simulink model "deadReckoning_rover_closedloop_mc40"  (R2023a)
settings: Solver=FixedStepAuto  StartTime=0.0  StopTime=inf  FixedStep=0.01  RelTol=1e-3  EnableMultiTasking=on
PreLoadFcn:
  | robotParameters;
model workspace (MAT data in the model file):
  axleLength = 0.085
  ticksPerRot = 1200
  wheelR = 0.045
undefined symbols (not defined in the file): DiscIntNeverNeededParam
libraries: M5Core_Library x4, simulink x1
settings Model: ExtModeTrigDuration=2  Creator=sseshadr  LastModifiedBy=auw_a
settings SolverCC: AlgebraicLoopSolver=TrustRegion
settings DataIOCC: ReturnWorkspaceOutputs=off
settings OptimizationCC: MaxStackSize=64  EfficientTunableParamExpr=on
settings DebuggingCC: ParameterPrecisionLossMsg=none  ParameterTunabilityLossMsg=error  UnconnectedInputMsg=warning  UnconnectedOutputMsg=warning  UnconnectedLineMsg=warning  ArithmeticOperatorsInVariantConditions=warning
settings HardwareCC: ProdBitPerPointer=32  ProdBitPerSizeT=32  ProdBitPerPtrDiffT=32  ProdLargestAtomicInteger=Long  ProdLargestAtomicFloat=Double  ProdWordSize=32  ProdHWDeviceType=ARM Compatible->ARM Cortex
settings ModelReferenceCC: EnableRefExpFcnMdlSchedulingChecks=on
settings SFSimCC: SimUseLocalCustomCode=off  MATLABDynamicMemAlloc=off  CustomCodeUndefinedFunction=UseInterfaceOnly
settings RTWCC: Description=Embedded Coder  SystemTargetFile=ert.tlc  HardwareBoard=ESP32-WROOM(Arduino Compatible)  TLCOptions="-aInlineSetEventsForThisBaseRateFcn=TLC_FALSE -aSuppressMultiTaskScheduler=TLC_FALSE    -aRateBasedStepFcn=0"  TemplateMakefile=ert_default_tmf  GenerateReport=on  RTWUseLocalCustomCode=off  Toolchain=ESP32  BuildConfiguration=Faster Runs  IncludeHyperlinkInReport=on  GenerateTraceInfo=on  GenerateTraceReport=on  GenerateTraceReportSl=on  GenerateTraceReportSf=on  GenerateTraceReportEml=on  DLArmComputeVersion=19.05
settings CodeAppCC: ForceParamTrailComments=on  IgnoreCustomStorageClasses=off  OperatorAnnotations=on  SimulinkDataObjDesc=on  SFDataObjDesc=on  MATLABFcnDesc=on  InsertBlockDesc=on  StateflowObjectComments=on  MATLABSourceComments=on
settings ERTTargetCC: MultiwordLength=2048  SupportContinuousTime=on  SupportVariableSizeSignals=on  ExtModeTransport=2  ExtModeStaticAlloc=on  ExtModeAutomaticAllocSize=off  ExtModeStaticAllocSize=65536  ExtModeMexFile=ext_xcp  ExtModeIntrfLevel=Level2 - Open

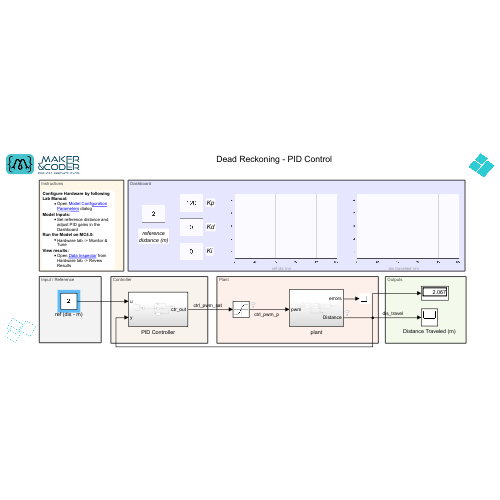
[thumbnail: Simulink's stored preview of the top-level diagram]
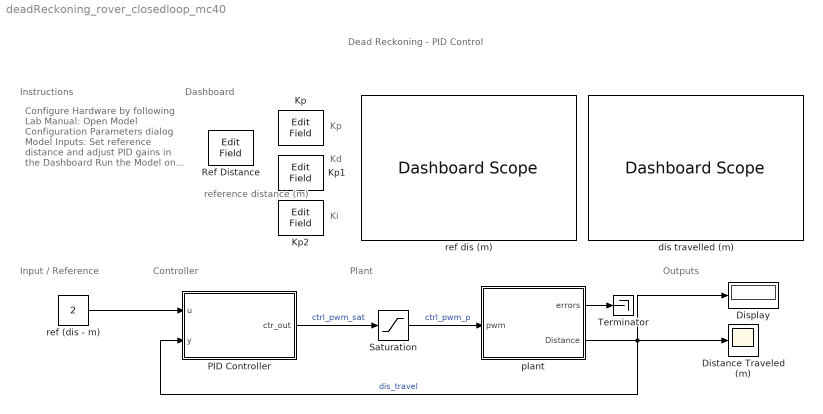
== system deadReckoning_rover_closedloop_mc40 ==
  note: Kp
  note: reference
      | distance (m)
  note: Dashboard
  note: Outputs
  note: Plant
  note: Controller
  note: Input / Reference
  note: Dead Reckoning - PID Control
  note: Kd
  note: Ki
  note: Configure Hardware by following Lab Manual:
      | Open Model Configuration Parameters dialog
      | Model Inputs:
      | Set reference distance and adjust PID gains in the Dashboard
      | Run the Model on MC4.0:
      | Hardware tab -> Monitor & Tune
      | View results:
      | Open Data Inspector from Hardware tab -> Revew Results
  note: Instructions
  Display : Display
  Distance Traveled (m) : Scope
  Kp : EditField  LabelPosition=Hide  ShowInitialText=on  Alignment=Center
  Kp1 : EditField  LabelPosition=Hide  ShowInitialText=on  Alignment=Center
  Kp2 : EditField  LabelPosition=Hide  ShowInitialText=on  Alignment=Center
  PID Controller : Subsystem
  Ref Distance : EditField  LabelPosition=Hide  ShowInitialText=on  Alignment=Center
  Saturation : Saturate  UpperLimit=127  LowerLimit=-127
  Terminator : Terminator
  dis travelled (m) : DashboardScope  Ymin=-5  Ymax=5  UpdateMode=Scroll
  plant : Subsystem
  ref (dis - m) : Constant  Value=2
  ref dis (m) : DashboardScope  Ymin=-5  Ymax=5  UpdateMode=Scroll
  wires:
  Saturation/1 -> plant/1(pwm)  "ctrl_pwm_p"
  plant/2(Distance) -> PID Controller/2(y), Distance Traveled (m)/1, Display/1  "dis_travel"
  ref (dis - m)/1 -> PID Controller/1(u)
  plant/1(errors) -> Terminator/1
  PID Controller/1(ctr_out) -> Saturation/1  "ctrl_pwm_sat"

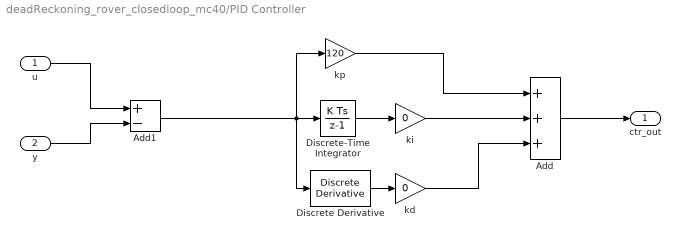
== system deadReckoning_rover_closedloop_mc40/PID Controller ==
  u : Inport
  y : Inport  Port=2
  Add : Sum  Inputs=+++
  Add1 : Sum  Inputs=+-
  Discrete Derivative : simulink/Discrete/Discrete Derivative  gainval=1.0  ICPrevScaledInput=0.0  OutMin=[]  OutMax=[]  OutDataType=fixdt(1, 16)  OutScaling=2^-10  DoSatur=off
  Discrete-Time Integrator : DiscreteIntegrator  SampleTime=-1  ICPrevOutput=DiscIntNeverNeededParam  ICPrevScaledInput=DiscIntNeverNeededParam
  kd : Gain  Gain=0
  ki : Gain  Gain=0
  kp : Gain  Gain=120
  ctr_out : Outport
  wires:
  kp/1 -> Add/1
  kd/1 -> Add/3
  Discrete-Time Integrator/1 -> ki/1
  Add1/1 -> Discrete Derivative/1, Discrete-Time Integrator/1, kp/1
  Discrete Derivative/1 -> kd/1
  ki/1 -> Add/2
  Add/1 -> ctr_out/1
  u/1 -> Add1/1
  y/1 -> Add1/2

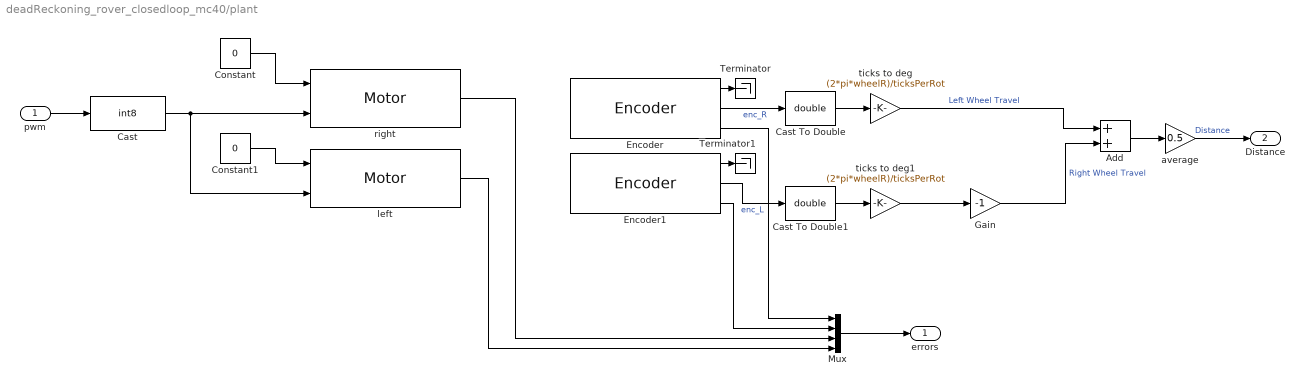
== system deadReckoning_rover_closedloop_mc40/plant ==
  pwm : Inport
  Add : Sum
  Cast : DataTypeConversion  OutDataTypeStr=int8  SaturateOnIntegerOverflow=off  RndMeth=Floor
  Cast To Double : DataTypeConversion  OutDataTypeStr=double  SaturateOnIntegerOverflow=off  RndMeth=Floor
  Cast To Double1 : DataTypeConversion  OutDataTypeStr=double  SaturateOnIntegerOverflow=off  RndMeth=Floor
  Constant : Constant  Value=0
  Constant1 : Constant  Value=0
  Encoder : M5Core_Library/Encoder  M5_motor=2  s=0.01
      link override encoder I2C Read: RegisterAddress=uint8(hex2dec('40')) + m  SlaveDataType=int8
  Encoder1 : M5Core_Library/Encoder  M5_motor=1  s=0.01
  Gain : Gain  Gain=-1
  Mux : Mux
  Terminator : Terminator
  Terminator1 : Terminator
  average : Gain  Gain=0.5
  left : M5Core_Library/Motor  M5_motor=M1
  right : M5Core_Library/Motor  M5_motor=M2
  ticks to deg : Gain  Gain=(2*pi*wheelR)/ticksPerRot
  ticks to deg1 : Gain  Gain=(2*pi*wheelR)/ticksPerRot
  errors : Outport
  Distance : Outport  Port=2
  wires:
  Mux/1 -> errors/1
  Encoder/2 -> Cast To Double/1  "enc_R"
  Constant/1 -> right/1
  Constant1/1 -> left/1
  pwm/1 -> Cast/1
  average/1 -> Distance/1  "Distance"
  Add/1 -> average/1
  ticks to deg/1 -> Add/1  "Left Wheel Travel"
  ticks to deg1/1 -> Gain/1
  Encoder1/2 -> Cast To Double1/1  "enc_L"
  Encoder/3 -> Mux/1
  Encoder1/3 -> Mux/2
  right/1 -> Mux/3
  left/1 -> Mux/4
  Encoder/1 -> Terminator/1
  Encoder1/1 -> Terminator1/1
  Gain/1 -> Add/2  "Right Wheel Travel"
  Cast To Double/1 -> ticks to deg/1
  Cast To Double1/1 -> ticks to deg1/1
  Cast/1 -> right/2, left/2
